simulink model "subsystemEquation"  (R2022b)
settings: Solver=VariableStepAuto  StartTime=0.0  StopTime=10.0  RelTol=1e-3
settings Model: Creator=Soliman Rabie  LastModifiedBy=Soliman Rabie

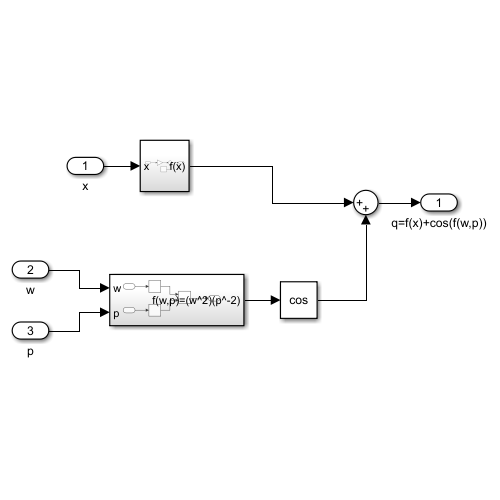
[thumbnail: Simulink's stored preview of the top-level diagram]
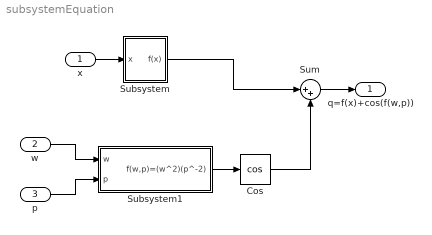
== system subsystemEquation ==
  x : Inport
  w : Inport  Port=2
  p : Inport  Port=3
  Cos : Trigonometry  Operator=cos
  Subsystem : Subsystem
  Subsystem1 : Subsystem
  Sum : Sum  Inputs=|++
  q=f(x)+cos(f(w,p)) : Outport
  wires:
  x/1 -> Subsystem/1(x)
  w/1 -> Subsystem1/1(w)
  p/1 -> Subsystem1/2(p)
  Subsystem1/1(f(w,p)=(w^2)(p^-2)) -> Cos/1
  Subsystem/1(f(x)) -> Sum/1
  Cos/1 -> Sum/2
  Sum/1 -> q=f(x)+cos(f(w,p))/1

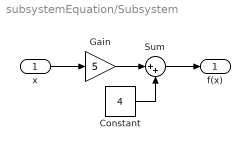
== system subsystemEquation/Subsystem ==
  x : Inport
  Constant : Constant  Value=4
  Gain : Gain  Gain=5
  Sum : Sum  Inputs=|++
  f(x) : Outport
  wires:
  Gain/1 -> Sum/1
  Sum/1 -> f(x)/1
  Constant/1 -> Sum/2
  x/1 -> Gain/1

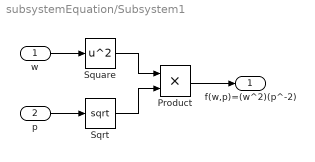
== system subsystemEquation/Subsystem1 ==
  w : Inport
  p : Inport  Port=2
  Product : Product
  Sqrt : Sqrt
  Square : Math  Operator=square
  f(w,p)=(w^2)(p^-2) : Outport
  wires:
  Product/1 -> f(w,p)=(w^2)(p^-2)/1
  w/1 -> Square/1
  Square/1 -> Product/1
  p/1 -> Sqrt/1
  Sqrt/1 -> Product/2
